simulink model "SimForces2020a"  (R2020a)
settings: Solver=daessc  StartTime=0.0  StopTime=10  FixedStep=0.001  RelTol=1e-4
values from neighbouring files (symbols this model uses):
  Bc1_V = [0;0;0;0;0;0]    [initializeSimulationGP.m]
  D22F = [0;0;0;0;0;0]    [initializeSimulationGP.m]
  filtDV = init2ndOrderLowPassFilter(35*2*pi,1,controller.dT)    [initializeLowPassFilters.m]
  filtEnc = init2ndOrderLowPassFilter(35*2*pi,1,controller.dT)    [initializeLowPassFilters.m]
undefined symbols (not defined in the file or in its folder): aux, B11_r_B11Tc1, B11_V, B11Ftot, B12_r_B12Tc2, B12_Rot_Tc2, B12_U_Tc2, B12_V, B12Ftot, B31_r_B31B41, B31_V, B31FTot, B32_r_B32B42, B32_Rot_B42, B32_U_B42, B32_V, B32FTot, B41_r_B41Tc1, B41_V, B41FTot, B42_r_B42Tc2, B42_Rot_Tc2, B42_U_Tc2, B42_V, B42FTot, B52_r_B52P32, B52_Rot_P32, B52_U_P32, B52_V, B52Ftot, Bc1_r_Bc1B11, Bc1_r_Bc1B31, Bc1FTot, Bc2_r_Bc2B12, Bc2_r_Bc2B32, Bc2_Rot_B12, Bc2_Rot_B32, Bc2_U_B12, Bc2_U_B32, Bc2_V, Bc2Tot, cmdMotion, controller, cyl1, cyl2, D22_V, dq1, dq11, dq12, dq2, dq21, dq22, dx1, dx2, dxt2, fc1, fc1r, fc2, fc2r, fct2 ... (+62)
libraries: sm_lib x31, nesl_utility x10
(part 4 of 7)

== system SimForces2020a/sbVDCController/sbFormTotalRequiredForces/sbTotalRequiredForcesRS1/sbFilteredVelocityDerivativeB11 ==
  u : Inport
  Demux : Demux  Outputs=6
  Mux : Mux  Inputs=6
  sbDiscreteDerivative1 : Subsystem
  sbDiscreteDerivative2 : Subsystem
  sbDiscreteDerivative3 : Subsystem
  sbDiscreteDerivative4 : Subsystem
  sbDiscreteDerivative5 : Subsystem
  sbDiscreteDerivative6 : Subsystem
  sbLowPassFilter1 : Subsystem
  sbLowPassFilter2 : Subsystem
  sbLowPassFilter3 : Subsystem
  sbLowPassFilter4 : Subsystem
  sbLowPassFilter5 : Subsystem
  sbLowPassFilter6 : Subsystem
  du : Outport
  wires:
  sbLowPassFilter5/1(dVFilt) -> Mux/5
  sbDiscreteDerivative4/1(du/dt) -> sbLowPassFilter4/1(dV)
  sbLowPassFilter4/1(dVFilt) -> Mux/4
  sbLowPassFilter3/1(dVFilt) -> Mux/3
  sbDiscreteDerivative3/1(du/dt) -> sbLowPassFilter3/1(dV)
  sbDiscreteDerivative2/1(du/dt) -> sbLowPassFilter2/1(dV)
  sbLowPassFilter6/1(dVFilt) -> Mux/6
  sbDiscreteDerivative6/1(du/dt) -> sbLowPassFilter6/1(dV)
  sbLowPassFilter1/1(dVFilt) -> Mux/1
  u/1 -> Demux/1
  Demux/2 -> sbDiscreteDerivative2/1(u)
  Demux/5 -> sbDiscreteDerivative5/1(u)
  sbDiscreteDerivative1/1(du/dt) -> sbLowPassFilter1/1(dV)
  Demux/6 -> sbDiscreteDerivative6/1(u)
  sbLowPassFilter2/1(dVFilt) -> Mux/2
  Demux/1 -> sbDiscreteDerivative1/1(u)
  Demux/4 -> sbDiscreteDerivative4/1(u)
  Mux/1 -> du/1
  sbDiscreteDerivative5/1(du/dt) -> sbLowPassFilter5/1(dV)
  Demux/3 -> sbDiscreteDerivative3/1(u)

== system SimForces2020a/sbVDCController/sbFormTotalRequiredForces/sbTotalRequiredForcesRS1/sbFilteredVelocityDerivativeB31 ==
  u : Inport
  Demux : Demux  Outputs=6
  Mux : Mux  Inputs=6
  sbDiscreteDerivative1 : Subsystem
  sbDiscreteDerivative2 : Subsystem
  sbDiscreteDerivative3 : Subsystem
  sbDiscreteDerivative4 : Subsystem
  sbDiscreteDerivative5 : Subsystem
  sbDiscreteDerivative6 : Subsystem
  sbLowPassFilter1 : Subsystem
  sbLowPassFilter2 : Subsystem
  sbLowPassFilter3 : Subsystem
  sbLowPassFilter4 : Subsystem
  sbLowPassFilter5 : Subsystem
  sbLowPassFilter6 : Subsystem
  du : Outport
  wires:
  Demux/3 -> sbDiscreteDerivative3/1(u)
  sbDiscreteDerivative5/1(du/dt) -> sbLowPassFilter5/1(dV)
  Mux/1 -> du/1
  Demux/4 -> sbDiscreteDerivative4/1(u)
  Demux/1 -> sbDiscreteDerivative1/1(u)
  sbLowPassFilter2/1(dVFilt) -> Mux/2
  Demux/6 -> sbDiscreteDerivative6/1(u)
  sbDiscreteDerivative1/1(du/dt) -> sbLowPassFilter1/1(dV)
  Demux/5 -> sbDiscreteDerivative5/1(u)
  Demux/2 -> sbDiscreteDerivative2/1(u)
  u/1 -> Demux/1
  sbLowPassFilter1/1(dVFilt) -> Mux/1
  sbDiscreteDerivative6/1(du/dt) -> sbLowPassFilter6/1(dV)
  sbLowPassFilter6/1(dVFilt) -> Mux/6
  sbDiscreteDerivative2/1(du/dt) -> sbLowPassFilter2/1(dV)
  sbDiscreteDerivative3/1(du/dt) -> sbLowPassFilter3/1(dV)
  sbLowPassFilter3/1(dVFilt) -> Mux/3
  sbLowPassFilter4/1(dVFilt) -> Mux/4
  sbDiscreteDerivative4/1(du/dt) -> sbLowPassFilter4/1(dV)
  sbLowPassFilter5/1(dVFilt) -> Mux/5

== system SimForces2020a/sbVDCController/sbFormTotalRequiredForces/sbTotalRequiredForcesRS1/sbFilteredVelocityDerivativeB41 ==
  u : Inport
  Demux : Demux  Outputs=6
  Mux : Mux  Inputs=6
  sbDiscreteDerivative1 : Subsystem
  sbDiscreteDerivative2 : Subsystem
  sbDiscreteDerivative3 : Subsystem
  sbDiscreteDerivative4 : Subsystem
  sbDiscreteDerivative5 : Subsystem
  sbDiscreteDerivative6 : Subsystem
  sbLowPassFilter1 : Subsystem
  sbLowPassFilter2 : Subsystem
  sbLowPassFilter3 : Subsystem
  sbLowPassFilter4 : Subsystem
  sbLowPassFilter5 : Subsystem
  sbLowPassFilter6 : Subsystem
  du : Outport
  wires:
  Demux/3 -> sbDiscreteDerivative3/1(u)
  sbDiscreteDerivative5/1(du/dt) -> sbLowPassFilter5/1(dV)
  Mux/1 -> du/1
  Demux/4 -> sbDiscreteDerivative4/1(u)
  Demux/1 -> sbDiscreteDerivative1/1(u)
  sbLowPassFilter2/1(dVFilt) -> Mux/2
  Demux/6 -> sbDiscreteDerivative6/1(u)
  sbDiscreteDerivative1/1(du/dt) -> sbLowPassFilter1/1(dV)
  Demux/5 -> sbDiscreteDerivative5/1(u)
  Demux/2 -> sbDiscreteDerivative2/1(u)
  u/1 -> Demux/1
  sbLowPassFilter1/1(dVFilt) -> Mux/1
  sbDiscreteDerivative6/1(du/dt) -> sbLowPassFilter6/1(dV)
  sbLowPassFilter6/1(dVFilt) -> Mux/6
  sbDiscreteDerivative2/1(du/dt) -> sbLowPassFilter2/1(dV)
  sbDiscreteDerivative3/1(du/dt) -> sbLowPassFilter3/1(dV)
  sbLowPassFilter3/1(dVFilt) -> Mux/3
  sbLowPassFilter4/1(dVFilt) -> Mux/4
  sbDiscreteDerivative4/1(du/dt) -> sbLowPassFilter4/1(dV)
  sbLowPassFilter5/1(dVFilt) -> Mux/5

== system SimForces2020a/sbVDCController/sbFormTotalRequiredForces/sbTotalRequiredForcesRS1/sbFilteredVelocityDerivativeBc1 ==
  u : Inport
  Demux : Demux  Outputs=6
  Mux : Mux  Inputs=6
  sbDiscreteDerivative1 : Subsystem
  sbDiscreteDerivative2 : Subsystem
  sbDiscreteDerivative3 : Subsystem
  sbDiscreteDerivative4 : Subsystem
  sbDiscreteDerivative5 : Subsystem
  sbDiscreteDerivative6 : Subsystem
  sbLowPassFilter1 : Subsystem
  sbLowPassFilter2 : Subsystem
  sbLowPassFilter3 : Subsystem
  sbLowPassFilter4 : Subsystem
  sbLowPassFilter5 : Subsystem
  sbLowPassFilter6 : Subsystem
  du : Outport
  wires:
  sbLowPassFilter5/1(dVFilt) -> Mux/5
  sbDiscreteDerivative4/1(du/dt) -> sbLowPassFilter4/1(dV)
  sbLowPassFilter4/1(dVFilt) -> Mux/4
  sbLowPassFilter3/1(dVFilt) -> Mux/3
  sbDiscreteDerivative3/1(du/dt) -> sbLowPassFilter3/1(dV)
  sbDiscreteDerivative2/1(du/dt) -> sbLowPassFilter2/1(dV)
  sbLowPassFilter6/1(dVFilt) -> Mux/6
  sbDiscreteDerivative6/1(du/dt) -> sbLowPassFilter6/1(dV)
  sbLowPassFilter1/1(dVFilt) -> Mux/1
  u/1 -> Demux/1
  Demux/2 -> sbDiscreteDerivative2/1(u)
  Demux/5 -> sbDiscreteDerivative5/1(u)
  sbDiscreteDerivative1/1(du/dt) -> sbLowPassFilter1/1(dV)
  Demux/6 -> sbDiscreteDerivative6/1(u)
  sbLowPassFilter2/1(dVFilt) -> Mux/2
  Demux/1 -> sbDiscreteDerivative1/1(u)
  Demux/4 -> sbDiscreteDerivative4/1(u)
  Mux/1 -> du/1
  sbDiscreteDerivative5/1(du/dt) -> sbLowPassFilter5/1(dV)
  Demux/3 -> sbDiscreteDerivative3/1(u)

== system SimForces2020a/sbVDCController/sbFormTotalRequiredForces/sbTotalRequiredForcesRS2/sbFilteredVelocityDerivativeB12 ==
  u : Inport
  Demux : Demux  Outputs=6
  Mux : Mux  Inputs=6
  sbDiscreteDerivative1 : Subsystem
  sbDiscreteDerivative2 : Subsystem
  sbDiscreteDerivative3 : Subsystem
  sbDiscreteDerivative4 : Subsystem
  sbDiscreteDerivative5 : Subsystem
  sbDiscreteDerivative6 : Subsystem
  sbLowPassFilter1 : Subsystem
  sbLowPassFilter2 : Subsystem
  sbLowPassFilter3 : Subsystem
  sbLowPassFilter4 : Subsystem
  sbLowPassFilter5 : Subsystem
  sbLowPassFilter6 : Subsystem
  du : Outport
  wires:
  Demux/3 -> sbDiscreteDerivative3/1(u)
  sbDiscreteDerivative5/1(du/dt) -> sbLowPassFilter5/1(dV)
  Mux/1 -> du/1
  Demux/4 -> sbDiscreteDerivative4/1(u)
  Demux/1 -> sbDiscreteDerivative1/1(u)
  sbLowPassFilter2/1(dVFilt) -> Mux/2
  Demux/6 -> sbDiscreteDerivative6/1(u)
  sbDiscreteDerivative1/1(du/dt) -> sbLowPassFilter1/1(dV)
  Demux/5 -> sbDiscreteDerivative5/1(u)
  Demux/2 -> sbDiscreteDerivative2/1(u)
  u/1 -> Demux/1
  sbLowPassFilter1/1(dVFilt) -> Mux/1
  sbDiscreteDerivative6/1(du/dt) -> sbLowPassFilter6/1(dV)
  sbLowPassFilter6/1(dVFilt) -> Mux/6
  sbDiscreteDerivative2/1(du/dt) -> sbLowPassFilter2/1(dV)
  sbDiscreteDerivative3/1(du/dt) -> sbLowPassFilter3/1(dV)
  sbLowPassFilter3/1(dVFilt) -> Mux/3
  sbLowPassFilter4/1(dVFilt) -> Mux/4
  sbDiscreteDerivative4/1(du/dt) -> sbLowPassFilter4/1(dV)
  sbLowPassFilter5/1(dVFilt) -> Mux/5

== system SimForces2020a/sbVDCController/sbFormTotalRequiredForces/sbTotalRequiredForcesRS2/sbFilteredVelocityDerivativeB32 ==
  u : Inport
  Demux : Demux  Outputs=6
  Mux : Mux  Inputs=6
  sbDiscreteDerivative1 : Subsystem
  sbDiscreteDerivative2 : Subsystem
  sbDiscreteDerivative3 : Subsystem
  sbDiscreteDerivative4 : Subsystem
  sbDiscreteDerivative5 : Subsystem
  sbDiscreteDerivative6 : Subsystem
  sbLowPassFilter1 : Subsystem
  sbLowPassFilter2 : Subsystem
  sbLowPassFilter3 : Subsystem
  sbLowPassFilter4 : Subsystem
  sbLowPassFilter5 : Subsystem
  sbLowPassFilter6 : Subsystem
  du : Outport
  wires:
  Demux/3 -> sbDiscreteDerivative3/1(u)
  sbDiscreteDerivative5/1(du/dt) -> sbLowPassFilter5/1(dV)
  Mux/1 -> du/1
  Demux/4 -> sbDiscreteDerivative4/1(u)
  Demux/1 -> sbDiscreteDerivative1/1(u)
  sbLowPassFilter2/1(dVFilt) -> Mux/2
  Demux/6 -> sbDiscreteDerivative6/1(u)
  sbDiscreteDerivative1/1(du/dt) -> sbLowPassFilter1/1(dV)
  Demux/5 -> sbDiscreteDerivative5/1(u)
  Demux/2 -> sbDiscreteDerivative2/1(u)
  u/1 -> Demux/1
  sbLowPassFilter1/1(dVFilt) -> Mux/1
  sbDiscreteDerivative6/1(du/dt) -> sbLowPassFilter6/1(dV)
  sbLowPassFilter6/1(dVFilt) -> Mux/6
  sbDiscreteDerivative2/1(du/dt) -> sbLowPassFilter2/1(dV)
  sbDiscreteDerivative3/1(du/dt) -> sbLowPassFilter3/1(dV)
  sbLowPassFilter3/1(dVFilt) -> Mux/3
  sbLowPassFilter4/1(dVFilt) -> Mux/4
  sbDiscreteDerivative4/1(du/dt) -> sbLowPassFilter4/1(dV)
  sbLowPassFilter5/1(dVFilt) -> Mux/5

== system SimForces2020a/sbVDCController/sbFormTotalRequiredForces/sbTotalRequiredForcesRS2/sbFilteredVelocityDerivativeB42 ==
  u : Inport
  Demux : Demux  Outputs=6
  Mux : Mux  Inputs=6
  sbDiscreteDerivative1 : Subsystem
  sbDiscreteDerivative2 : Subsystem
  sbDiscreteDerivative3 : Subsystem
  sbDiscreteDerivative4 : Subsystem
  sbDiscreteDerivative5 : Subsystem
  sbDiscreteDerivative6 : Subsystem
  sbLowPassFilter1 : Subsystem
  sbLowPassFilter2 : Subsystem
  sbLowPassFilter3 : Subsystem
  sbLowPassFilter4 : Subsystem
  sbLowPassFilter5 : Subsystem
  sbLowPassFilter6 : Subsystem
  du : Outport
  wires:
  Demux/3 -> sbDiscreteDerivative3/1(u)
  sbDiscreteDerivative5/1(du/dt) -> sbLowPassFilter5/1(dV)
  Mux/1 -> du/1
  Demux/4 -> sbDiscreteDerivative4/1(u)
  Demux/1 -> sbDiscreteDerivative1/1(u)
  sbLowPassFilter2/1(dVFilt) -> Mux/2
  Demux/6 -> sbDiscreteDerivative6/1(u)
  sbDiscreteDerivative1/1(du/dt) -> sbLowPassFilter1/1(dV)
  Demux/5 -> sbDiscreteDerivative5/1(u)
  Demux/2 -> sbDiscreteDerivative2/1(u)
  u/1 -> Demux/1
  sbLowPassFilter1/1(dVFilt) -> Mux/1
  sbDiscreteDerivative6/1(du/dt) -> sbLowPassFilter6/1(dV)
  sbLowPassFilter6/1(dVFilt) -> Mux/6
  sbDiscreteDerivative2/1(du/dt) -> sbLowPassFilter2/1(dV)
  sbDiscreteDerivative3/1(du/dt) -> sbLowPassFilter3/1(dV)
  sbLowPassFilter3/1(dVFilt) -> Mux/3
  sbLowPassFilter4/1(dVFilt) -> Mux/4
  sbDiscreteDerivative4/1(du/dt) -> sbLowPassFilter4/1(dV)
  sbLowPassFilter5/1(dVFilt) -> Mux/5

== system SimForces2020a/sbVDCController/sbFormTotalRequiredForces/sbTotalRequiredForcesRS2/sbFilteredVelocityDerivativeBc2 ==
  u : Inport
  Demux : Demux  Outputs=6
  Mux : Mux  Inputs=6
  sbDiscreteDerivative1 : Subsystem
  sbDiscreteDerivative2 : Subsystem
  sbDiscreteDerivative3 : Subsystem
  sbDiscreteDerivative4 : Subsystem
  sbDiscreteDerivative5 : Subsystem
  sbDiscreteDerivative6 : Subsystem
  sbLowPassFilter1 : Subsystem
  sbLowPassFilter2 : Subsystem
  sbLowPassFilter3 : Subsystem
  sbLowPassFilter4 : Subsystem
  sbLowPassFilter5 : Subsystem
  sbLowPassFilter6 : Subsystem
  du : Outport
  wires:
  Demux/3 -> sbDiscreteDerivative3/1(u)
  sbDiscreteDerivative5/1(du/dt) -> sbLowPassFilter5/1(dV)
  Mux/1 -> du/1
  Demux/4 -> sbDiscreteDerivative4/1(u)
  Demux/1 -> sbDiscreteDerivative1/1(u)
  sbLowPassFilter2/1(dVFilt) -> Mux/2
  Demux/6 -> sbDiscreteDerivative6/1(u)
  sbDiscreteDerivative1/1(du/dt) -> sbLowPassFilter1/1(dV)
  Demux/5 -> sbDiscreteDerivative5/1(u)
  Demux/2 -> sbDiscreteDerivative2/1(u)
  u/1 -> Demux/1
  sbLowPassFilter1/1(dVFilt) -> Mux/1
  sbDiscreteDerivative6/1(du/dt) -> sbLowPassFilter6/1(dV)
  sbLowPassFilter6/1(dVFilt) -> Mux/6
  sbDiscreteDerivative2/1(du/dt) -> sbLowPassFilter2/1(dV)
  sbDiscreteDerivative3/1(du/dt) -> sbLowPassFilter3/1(dV)
  sbLowPassFilter3/1(dVFilt) -> Mux/3
  sbLowPassFilter4/1(dVFilt) -> Mux/4
  sbDiscreteDerivative4/1(du/dt) -> sbLowPassFilter4/1(dV)
  sbLowPassFilter5/1(dVFilt) -> Mux/5

== system SimForces2020a/sbVDCController/sbFormAnalyticQuantities/sbPrismaticSegment2/sbGeomPropPS2/sbDiscreteDerivative ==
  u : Inport
  Add : Sum  Inputs=-+
  Gain6 : Gain  Gain=1/(2*controller.dT)
  Integer Delay : Delay  InitialConditionSource=Input port  InitialCondition=0  SampleTime=controller.dT
      settings: InputPortMap=u0,p4
  du/dt : Outport  PortDimensions=1
  wires:
  u/1 -> Integer Delay/1, Integer Delay/2, Add/2
  Gain6/1 -> du/dt/1
  Integer Delay/1 -> Add/1
  Add/1 -> Gain6/1

== system SimForces2020a/sbVDCController/sbFormAnalyticQuantities/sbRevoluteSegment1/sbGeomPropRS1/sbLiftPistonStroke ==
  note: Get inputs...
  note: Process data...
  note: Pass to outputs...
  q1 : Inport  Unit=rad  PortDimensions=1
  liftPistonStroke : MATLAB Function  TreatAsAtomicUnit=on
  x1 : Outport  Unit=m  PortDimensions=1
  wires:
  [x1] -> x1/1  "x1"
  liftPistonStroke/1(x1) -> [x1]  "x1"
  [q1] -> liftPistonStroke/1(q1)  "q1"
  q1/1 -> [q1]  "q1"

== system SimForces2020a/sbVDCController/sbFormAnalyticQuantities/sbRevoluteSegment1/sbGeomPropRS1/sbLiftPistonVelocity ==
  note: Get inputs...
  note: Process data...
  note: Pass to output...
  dq1 : Inport
  x1 : Inport  Port=2
  q1 : Inport  Port=3
  liftPistonVelocity : MATLAB Function  TreatAsAtomicUnit=on
  dx1 : Outport
  wires:
  [dx1] -> dx1/1  "dx1"
  liftPistonVelocity/1(dx1) -> [dx1]  "dx1"
  [q1] -> liftPistonVelocity/3(q1)  "q1"
  q1/1 -> [q1]  "q1"
  [x1] -> liftPistonVelocity/2(x1)  "x1"
  x1/1 -> [x1]  "x1"
  [dq1] -> liftPistonVelocity/1(dq1)  "dq1"
  dq1/1 -> [dq1]  "dq1"

== system SimForces2020a/sbVDCController/sbFormAnalyticQuantities/sbRevoluteSegment1/sbGeomPropRS1/sbq11AngleValue ==
  note: Get inputs...
  note: Process data...
  note: Pass to outputs...
  x1 : Inport
  q11AngleValue : MATLAB Function  TreatAsAtomicUnit=on
  q11 : Outport
  wires:
  [q11] -> q11/1  "q11"
  q11AngleValue/1(q11) -> [q11]  "q11"
  [x1] -> q11AngleValue/1(x1)  "x1"
  x1/1 -> [x1]  "x1"

== system SimForces2020a/sbVDCController/sbFormAnalyticQuantities/sbRevoluteSegment1/sbGeomPropRS1/sbq11AngleVelocity ==
  note: Get inputs...
  note: Process data...
  note: Pass to outputs...
  x1 : Inport
  q11 : Inport  Port=2
  dx1 : Inport  Port=3
  q11AngleRate : MATLAB Function  TreatAsAtomicUnit=on
  dq11 : Outport
  wires:
  [dq11] -> dq11/1  "dq11"
  q11AngleRate/1(dq11) -> [dq11]  "dq11"
  [dx1] -> q11AngleRate/3(dx1)  "dx1"
  [q11] -> q11AngleRate/2(q11)  "q11"
  [x1] -> q11AngleRate/1(x1)  "x1"
  dx1/1 -> [dx1]  "dx1"
  q11/1 -> [q11]  "q11"
  x1/1 -> [x1]  "x1"

== system SimForces2020a/sbVDCController/sbFormAnalyticQuantities/sbRevoluteSegment1/sbGeomPropRS1/sbq12AngleRate ==
  note: Get inputs...
  note: Pass to outputs...
  note: Process data...
  x1 : Inport
  q12 : Inport  Port=2
  dx1 : Inport  Port=3
  q12AngleRate : MATLAB Function  TreatAsAtomicUnit=on
  dq12 : Outport
  wires:
  [dx1] -> q12AngleRate/3(dx1)  "dx1"
  [x1] -> q12AngleRate/1(x1)  "x1"
  [q12] -> q12AngleRate/2(q12)  "q12"
  x1/1 -> [x1]  "x1"
  q12AngleRate/1(dq12) -> [dq12]  "dq12"
  [dq12] -> dq12/1  "dq12"
  q12/1 -> [q12]  "q12"
  dx1/1 -> [dx1]  "dx1"

== system SimForces2020a/sbVDCController/sbFormAnalyticQuantities/sbRevoluteSegment1/sbGeomPropRS1/sbq12AngleValue ==
  note: Get inputs...
  note: Process data...
  note: Pass to outputs...
  x1 : Inport
  q12AngleValue : MATLAB Function  TreatAsAtomicUnit=on
  q12 : Outport
  wires:
  [q12] -> q12/1  "q12"
  q12AngleValue/1(q12) -> [q12]  "q12"
  [x1] -> q12AngleValue/1(x1)  "x1"
  x1/1 -> [x1]  "x1"

== system SimForces2020a/sbVDCController/sbFormAnalyticQuantities/sbRevoluteSegment1/sbGeomPropRS1/sbq1AngleRate ==
  note: Get inputs...
  note: Process data...
  note: Pass to outputs...
  q1 : Inport
  sbDiscreteDerivative : Subsystem
  dq1 : Outport
  wires:
  sbDiscreteDerivative/1(du/dt) -> [dq1]  "dq1"
  [dq1] -> dq1/1  "dq1"
  [q1] -> sbDiscreteDerivative/1(u)  "q1"
  q1/1 -> [q1]  "q1"

== system SimForces2020a/sbVDCController/sbFormAnalyticQuantities/sbRevoluteSegment2/sbGeomPropRS2/sbTiltPistonStroke ==
  note: Pass to outputs...
  note: Get inputs...
  note: Derive the tilt piston stroke from q2-angle value...
  note: Process data...
  q2 : Inport
  tiltPistonStroke : MATLAB Function  TreatAsAtomicUnit=on
  x2 : Outport
  wires:
  q2/1 -> [q2]  "q2"
  [x2] -> x2/1  "x2"
  tiltPistonStroke/1(x2) -> [x2]  "x2"
  [q2] -> tiltPistonStroke/1(q2)  "q2"

== system SimForces2020a/sbVDCController/sbFormAnalyticQuantities/sbRevoluteSegment2/sbGeomPropRS2/sbTiltPistonVelocity ==
  note: Get inputs...
  note: Process data...
  note: Pass to output...
  dq2 : Inport
  x2 : Inport  Port=2
  q2 : Inport  Port=3
  tiltPistonVelocity : MATLAB Function  TreatAsAtomicUnit=on
  dx2 : Outport
  wires:
  tiltPistonVelocity/1(dx2) -> [dx2]  "dx2"
  [dx2] -> dx2/1  "dx2"
  [q2] -> tiltPistonVelocity/3(q2)  "q2"
  q2/1 -> [q2]  "q2"
  [x2] -> tiltPistonVelocity/2(x2)  "x2"
  x2/1 -> [x2]  "x2"
  [dq2] -> tiltPistonVelocity/1(dq2)  "dq2"
  dq2/1 -> [dq2]  "dq2"

== system SimForces2020a/sbVDCController/sbFormAnalyticQuantities/sbRevoluteSegment2/sbGeomPropRS2/sbq21AngleRate ==
  note: Get inputs...
  note: Process data...
  note: Pass to outputs...
  x2 : Inport
  q21 : Inport  Port=2
  dx2 : Inport  Port=3
  q21AngleRate : MATLAB Function  TreatAsAtomicUnit=on
  dq21 : Outport
  wires:
  [q21] -> q21AngleRate/2(q21)  "q21"
  [dx2] -> q21AngleRate/3(dx2)  "dx2"
  [dq21] -> dq21/1  "dq21"
  q21AngleRate/1(dq21) -> [dq21]  "dq21"
  [x2] -> q21AngleRate/1(x2)  "x2"
  dx2/1 -> [dx2]  "dx2"
  q21/1 -> [q21]  "q21"
  x2/1 -> [x2]  "x2"

== system SimForces2020a/sbVDCController/sbFormAnalyticQuantities/sbRevoluteSegment2/sbGeomPropRS2/sbq21AngleValue ==
  note: Get inputs...
  note: Process data...
  note: Pass to outputs...
  x2 : Inport
  q21AngleValue : MATLAB Function  TreatAsAtomicUnit=on
  q21 : Outport
  wires:
  q21AngleValue/1(q21) -> [q21]  "q21"
  [x2] -> q21AngleValue/1(x2)  "x2"
  [q21] -> q21/1  "q21"
  x2/1 -> [x2]  "x2"

== system SimForces2020a/sbVDCController/sbFormAnalyticQuantities/sbRevoluteSegment2/sbGeomPropRS2/sbq22AngleRate ==
  note: Get inputs...
  note: Pass to outputs...
  note: Process data...
  x2 : Inport
  q22 : Inport  Port=2
  dx2 : Inport  Port=3
  q22AngleRate : MATLAB Function  TreatAsAtomicUnit=on
  dq22 : Outport
  wires:
  [x2] -> q22AngleRate/1(x2)  "x2"
  x2/1 -> [x2]  "x2"
  q22AngleRate/1(dq22) -> [dq22]  "dq22"
  [dq22] -> dq22/1  "dq22"
  q22/1 -> [q22]  "q22"
  dx2/1 -> [dx2]  "dx2"
  [q22] -> q22AngleRate/2(q22)  "q22"
  [dx2] -> q22AngleRate/3(dx2)  "dx2"

== system SimForces2020a/sbVDCController/sbFormAnalyticQuantities/sbRevoluteSegment2/sbGeomPropRS2/sbq22AngleValue ==
  note: Pass to outputs...
  note: Process data...
  note: Get inputs...
  x2 : Inport
  q22AngleValue : MATLAB Function  TreatAsAtomicUnit=on
  q22 : Outport
  wires:
  x2/1 -> [x2]  "x2"
  [x2] -> q22AngleValue/1(x2)  "x2"
  q22AngleValue/1(q22) -> [q22]  "q22"
  [q22] -> q22/1  "q22"

== system SimForces2020a/sbVDCController/sbFormAnalyticQuantities/sbRevoluteSegment2/sbGeomPropRS2/sbq2AngleRate ==
  note: Get inputs...
  note: Process data...
  note: Pass to outputs...
  q2 : Inport
  sbDiscreteDerivative : Subsystem
  dq2 : Outport
  wires:
  sbDiscreteDerivative/1(du/dt) -> [dq2]  "dq2"
  [dq2] -> dq2/1  "dq2"
  [q2] -> sbDiscreteDerivative/1(u)  "q2"
  q2/1 -> [q2]  "q2"

== system SimForces2020a/sbVDCController/sbFormTotalRequiredForces/sbTotalRequiredForcesPS2/sbFilteredVelocityDerivativeB52/sbDiscreteDerivative1 ==
  u : Inport
  Add : Sum  Inputs=-+
  Gain6 : Gain  Gain=1/(2*controller.dT)
  Integer Delay : Delay  InitialConditionSource=Input port  InitialCondition=0  SampleTime=controller.dT
      settings: InputPortMap=u0,p4
  du/dt : Outport  PortDimensions=1
  wires:
  Add/1 -> Gain6/1
  u/1 -> Integer Delay/1, Integer Delay/2, Add/2
  Integer Delay/1 -> Add/1
  Gain6/1 -> du/dt/1

== system SimForces2020a/sbVDCController/sbFormTotalRequiredForces/sbTotalRequiredForcesPS2/sbFilteredVelocityDerivativeB52/sbDiscreteDerivative2 ==
  u : Inport
  Add : Sum  Inputs=-+
  Gain6 : Gain  Gain=1/(2*controller.dT)
  Integer Delay : Delay  InitialConditionSource=Input port  InitialCondition=0  SampleTime=controller.dT
      settings: InputPortMap=u0,p4
  du/dt : Outport  PortDimensions=1
  wires:
  u/1 -> Integer Delay/1, Integer Delay/2, Add/2
  Integer Delay/1 -> Add/1
  Add/1 -> Gain6/1
  Gain6/1 -> du/dt/1

== system SimForces2020a/sbVDCController/sbFormTotalRequiredForces/sbTotalRequiredForcesPS2/sbFilteredVelocityDerivativeB52/sbDiscreteDerivative3 ==
  u : Inport
  Add : Sum  Inputs=-+
  Gain6 : Gain  Gain=1/(2*controller.dT)
  Integer Delay : Delay  InitialConditionSource=Input port  InitialCondition=0  SampleTime=controller.dT
      settings: InputPortMap=u0,p4
  du/dt : Outport  PortDimensions=1
  wires:
  Add/1 -> Gain6/1
  Integer Delay/1 -> Add/1
  u/1 -> Integer Delay/1, Integer Delay/2, Add/2
  Gain6/1 -> du/dt/1

== system SimForces2020a/sbVDCController/sbFormTotalRequiredForces/sbTotalRequiredForcesPS2/sbFilteredVelocityDerivativeB52/sbDiscreteDerivative4 ==
  u : Inport
  Add : Sum  Inputs=-+
  Gain6 : Gain  Gain=1/(2*controller.dT)
  Integer Delay : Delay  InitialConditionSource=Input port  InitialCondition=0  SampleTime=controller.dT
      settings: InputPortMap=u0,p4
  du/dt : Outport  PortDimensions=1
  wires:
  Add/1 -> Gain6/1
  Integer Delay/1 -> Add/1
  u/1 -> Integer Delay/1, Integer Delay/2, Add/2
  Gain6/1 -> du/dt/1

== system SimForces2020a/sbVDCController/sbFormTotalRequiredForces/sbTotalRequiredForcesPS2/sbFilteredVelocityDerivativeB52/sbDiscreteDerivative5 ==
  u : Inport
  Add : Sum  Inputs=-+
  Gain6 : Gain  Gain=1/(2*controller.dT)
  Integer Delay : Delay  InitialConditionSource=Input port  InitialCondition=0  SampleTime=controller.dT
      settings: InputPortMap=u0,p4
  du/dt : Outport  PortDimensions=1
  wires:
  Add/1 -> Gain6/1
  Integer Delay/1 -> Add/1
  u/1 -> Integer Delay/1, Integer Delay/2, Add/2
  Gain6/1 -> du/dt/1

== system SimForces2020a/sbVDCController/sbFormTotalRequiredForces/sbTotalRequiredForcesPS2/sbFilteredVelocityDerivativeB52/sbDiscreteDerivative6 ==
  u : Inport
  Add : Sum  Inputs=-+
  Gain6 : Gain  Gain=1/(2*controller.dT)
  Integer Delay : Delay  InitialConditionSource=Input port  InitialCondition=0  SampleTime=controller.dT
      settings: InputPortMap=u0,p4
  du/dt : Outport  PortDimensions=1
  wires:
  Add/1 -> Gain6/1
  Integer Delay/1 -> Add/1
  u/1 -> Integer Delay/1, Integer Delay/2, Add/2
  Gain6/1 -> du/dt/1

== system SimForces2020a/sbVDCController/sbFormTotalRequiredForces/sbTotalRequiredForcesPS2/sbFilteredVelocityDerivativeB52/sbLowPassFilter1 ==
  dV : Inport
  Delay : Delay  InitialConditionSource=Input port  SampleTime=filtDV.dT
      settings: InputPortMap=u0,p4
  Delay1 : Delay  DelayLength=1  InitialConditionSource=Input port  SampleTime=filtDV.dT
      settings: InputPortMap=u0,p4
  Delay2 : Delay  DelayLength=0  InitialConditionSource=Input port  SampleTime=filtDV.dT
      settings: InputPortMap=u0,p4
  Delay3 : Delay  InitialConditionSource=Input port  SampleTime=filtDV.dT
      settings: InputPortMap=u0,p4
  Delay4 : Delay  DelayLength=1  InitialConditionSource=Input port  SampleTime=filtDV.dT
      settings: InputPortMap=u0,p4
  Gain : Gain  Gain=filtDV.a0
  Gain1 : Gain  Gain=filtDV.b1
  Gain2 : Gain  Gain=filtDV.b2
  Gain3 : Gain  Gain=filtDV.b0
  Gain4 : Gain  Gain=filtDV.a1
  Sum : Sum  Inputs=|--+++
  dVFilt : Outport
  wires:
  Gain3/1 -> Sum/5
  Gain2/1 -> Sum/3
  Delay4/1 -> Gain4/1
  Delay/1 -> Gain/1
  Delay1/1 -> Gain1/1
  Delay2/1 -> Gain2/1
  Gain4/1 -> Sum/1
  Sum/1 -> dVFilt/1, Delay4/1, Delay/1  "dVFilt"
  dV/1 -> Delay2/1, Delay2/2, Delay1/1, Delay3/2, Delay3/1, Delay1/2, Delay4/2, Delay/2  "dV"
  Gain1/1 -> Sum/4
  Gain/1 -> Sum/2
  Delay3/1 -> Gain3/1

== system SimForces2020a/sbVDCController/sbFormTotalRequiredForces/sbTotalRequiredForcesPS2/sbFilteredVelocityDerivativeB52/sbLowPassFilter2 ==
  dV : Inport
  Delay : Delay  InitialConditionSource=Input port  SampleTime=filtDV.dT
      settings: InputPortMap=u0,p4
  Delay1 : Delay  DelayLength=1  InitialConditionSource=Input port  SampleTime=filtDV.dT
      settings: InputPortMap=u0,p4
  Delay2 : Delay  DelayLength=0  InitialConditionSource=Input port  SampleTime=filtDV.dT
      settings: InputPortMap=u0,p4
  Delay3 : Delay  InitialConditionSource=Input port  SampleTime=filtDV.dT
      settings: InputPortMap=u0,p4
  Delay4 : Delay  DelayLength=1  InitialConditionSource=Input port  SampleTime=filtDV.dT
      settings: InputPortMap=u0,p4
  Gain : Gain  Gain=filtDV.a0
  Gain1 : Gain  Gain=filtDV.b1
  Gain2 : Gain  Gain=filtDV.b2
  Gain3 : Gain  Gain=filtDV.b0
  Gain4 : Gain  Gain=filtDV.a1
  Sum : Sum  Inputs=|--+++
  dVFilt : Outport
  wires:
  Delay3/1 -> Gain3/1
  Gain/1 -> Sum/2
  Gain1/1 -> Sum/4
  dV/1 -> Delay/2, Delay4/2, Delay1/2, Delay3/1, Delay3/2, Delay1/1, Delay2/2, Delay2/1  "dV"
  Sum/1 -> Delay/1, Delay4/1, dVFilt/1  "dVFilt"
  Gain4/1 -> Sum/1
  Delay2/1 -> Gain2/1
  Delay1/1 -> Gain1/1
  Delay/1 -> Gain/1
  Delay4/1 -> Gain4/1
  Gain2/1 -> Sum/3
  Gain3/1 -> Sum/5

== system SimForces2020a/sbVDCController/sbFormTotalRequiredForces/sbTotalRequiredForcesPS2/sbFilteredVelocityDerivativeB52/sbLowPassFilter3 ==
  dV : Inport
  Delay : Delay  InitialConditionSource=Input port  SampleTime=filtDV.dT
      settings: InputPortMap=u0,p4
  Delay1 : Delay  DelayLength=1  InitialConditionSource=Input port  SampleTime=filtDV.dT
      settings: InputPortMap=u0,p4
  Delay2 : Delay  DelayLength=0  InitialConditionSource=Input port  SampleTime=filtDV.dT
      settings: InputPortMap=u0,p4
  Delay3 : Delay  InitialConditionSource=Input port  SampleTime=filtDV.dT
      settings: InputPortMap=u0,p4
  Delay4 : Delay  DelayLength=1  InitialConditionSource=Input port  SampleTime=filtDV.dT
      settings: InputPortMap=u0,p4
  Gain : Gain  Gain=filtDV.a0
  Gain1 : Gain  Gain=filtDV.b1
  Gain2 : Gain  Gain=filtDV.b2
  Gain3 : Gain  Gain=filtDV.b0
  Gain4 : Gain  Gain=filtDV.a1
  Sum : Sum  Inputs=|--+++
  dVFilt : Outport
  wires:
  Gain3/1 -> Sum/5
  Gain2/1 -> Sum/3
  Delay4/1 -> Gain4/1
  Delay/1 -> Gain/1
  Delay1/1 -> Gain1/1
  Delay2/1 -> Gain2/1
  Gain4/1 -> Sum/1
  Sum/1 -> dVFilt/1, Delay4/1, Delay/1  "dVFilt"
  dV/1 -> Delay2/1, Delay2/2, Delay1/1, Delay3/2, Delay3/1, Delay1/2, Delay4/2, Delay/2  "dV"
  Gain1/1 -> Sum/4
  Gain/1 -> Sum/2
  Delay3/1 -> Gain3/1

== system SimForces2020a/sbVDCController/sbFormTotalRequiredForces/sbTotalRequiredForcesPS2/sbFilteredVelocityDerivativeB52/sbLowPassFilter4 ==
  dV : Inport
  Delay : Delay  InitialConditionSource=Input port  SampleTime=filtDV.dT
      settings: InputPortMap=u0,p4
  Delay1 : Delay  DelayLength=1  InitialConditionSource=Input port  SampleTime=filtDV.dT
      settings: InputPortMap=u0,p4
  Delay2 : Delay  DelayLength=0  InitialConditionSource=Input port  SampleTime=filtDV.dT
      settings: InputPortMap=u0,p4
  Delay3 : Delay  InitialConditionSource=Input port  SampleTime=filtDV.dT
      settings: InputPortMap=u0,p4
  Delay4 : Delay  DelayLength=1  InitialConditionSource=Input port  SampleTime=filtDV.dT
      settings: InputPortMap=u0,p4
  Gain : Gain  Gain=filtDV.a0
  Gain1 : Gain  Gain=filtDV.b1
  Gain2 : Gain  Gain=filtDV.b2
  Gain3 : Gain  Gain=filtDV.b0
  Gain4 : Gain  Gain=filtDV.a1
  Sum : Sum  Inputs=|--+++
  dVFilt : Outport
  wires:
  Delay3/1 -> Gain3/1
  Gain/1 -> Sum/2
  Gain1/1 -> Sum/4
  dV/1 -> Delay/2, Delay4/2, Delay1/2, Delay3/1, Delay3/2, Delay1/1, Delay2/2, Delay2/1  "dV"
  Sum/1 -> Delay/1, Delay4/1, dVFilt/1  "dVFilt"
  Gain4/1 -> Sum/1
  Delay2/1 -> Gain2/1
  Delay1/1 -> Gain1/1
  Delay/1 -> Gain/1
  Delay4/1 -> Gain4/1
  Gain2/1 -> Sum/3
  Gain3/1 -> Sum/5

== system SimForces2020a/sbVDCController/sbFormTotalRequiredForces/sbTotalRequiredForcesPS2/sbFilteredVelocityDerivativeB52/sbLowPassFilter5 ==
  dV : Inport
  Delay : Delay  InitialConditionSource=Input port  SampleTime=filtDV.dT
      settings: InputPortMap=u0,p4
  Delay1 : Delay  DelayLength=1  InitialConditionSource=Input port  SampleTime=filtDV.dT
      settings: InputPortMap=u0,p4
  Delay2 : Delay  DelayLength=0  InitialConditionSource=Input port  SampleTime=filtDV.dT
      settings: InputPortMap=u0,p4
  Delay3 : Delay  InitialConditionSource=Input port  SampleTime=filtDV.dT
      settings: InputPortMap=u0,p4
  Delay4 : Delay  DelayLength=1  InitialConditionSource=Input port  SampleTime=filtDV.dT
      settings: InputPortMap=u0,p4
  Gain : Gain  Gain=filtDV.a0
  Gain1 : Gain  Gain=filtDV.b1
  Gain2 : Gain  Gain=filtDV.b2
  Gain3 : Gain  Gain=filtDV.b0
  Gain4 : Gain  Gain=filtDV.a1
  Sum : Sum  Inputs=|--+++
  dVFilt : Outport
  wires:
  Gain3/1 -> Sum/5
  Gain2/1 -> Sum/3
  Delay4/1 -> Gain4/1
  Delay/1 -> Gain/1
  Delay1/1 -> Gain1/1
  Delay2/1 -> Gain2/1
  Gain4/1 -> Sum/1
  Sum/1 -> dVFilt/1, Delay4/1, Delay/1  "dVFilt"
  dV/1 -> Delay2/1, Delay2/2, Delay1/1, Delay3/2, Delay3/1, Delay1/2, Delay4/2, Delay/2  "dV"
  Gain1/1 -> Sum/4
  Gain/1 -> Sum/2
  Delay3/1 -> Gain3/1

== system SimForces2020a/sbVDCController/sbFormTotalRequiredForces/sbTotalRequiredForcesPS2/sbFilteredVelocityDerivativeB52/sbLowPassFilter6 ==
  dV : Inport
  Delay : Delay  InitialConditionSource=Input port  SampleTime=filtDV.dT
      settings: InputPortMap=u0,p4
  Delay1 : Delay  DelayLength=1  InitialConditionSource=Input port  SampleTime=filtDV.dT
      settings: InputPortMap=u0,p4
  Delay2 : Delay  DelayLength=0  InitialConditionSource=Input port  SampleTime=filtDV.dT
      settings: InputPortMap=u0,p4
  Delay3 : Delay  InitialConditionSource=Input port  SampleTime=filtDV.dT
      settings: InputPortMap=u0,p4
  Delay4 : Delay  DelayLength=1  InitialConditionSource=Input port  SampleTime=filtDV.dT
      settings: InputPortMap=u0,p4
  Gain : Gain  Gain=filtDV.a0
  Gain1 : Gain  Gain=filtDV.b1
  Gain2 : Gain  Gain=filtDV.b2
  Gain3 : Gain  Gain=filtDV.b0
  Gain4 : Gain  Gain=filtDV.a1
  Sum : Sum  Inputs=|--+++
  dVFilt : Outport
  wires:
  Delay3/1 -> Gain3/1
  Gain/1 -> Sum/2
  Gain1/1 -> Sum/4
  dV/1 -> Delay/2, Delay4/2, Delay1/2, Delay3/1, Delay3/2, Delay1/1, Delay2/2, Delay2/1  "dV"
  Sum/1 -> Delay/1, Delay4/1, dVFilt/1  "dVFilt"
  Gain4/1 -> Sum/1
  Delay2/1 -> Gain2/1
  Delay1/1 -> Gain1/1
  Delay/1 -> Gain/1
  Delay4/1 -> Gain4/1
  Gain2/1 -> Sum/3
  Gain3/1 -> Sum/5

== system SimForces2020a/sbVDCController/sbFormTotalRequiredForces/sbTotalRequiredForcesPS2/sbFilteredVelocityDerivativeP22/sbDiscreteDerivative1 ==
  u : Inport
  Add : Sum  Inputs=-+
  Gain6 : Gain  Gain=1/(2*controller.dT)
  Integer Delay : Delay  InitialConditionSource=Input port  InitialCondition=0  SampleTime=controller.dT
      settings: InputPortMap=u0,p4
  du/dt : Outport  PortDimensions=1
  wires:
  Add/1 -> Gain6/1
  u/1 -> Integer Delay/1, Integer Delay/2, Add/2
  Integer Delay/1 -> Add/1
  Gain6/1 -> du/dt/1

== system SimForces2020a/sbVDCController/sbFormTotalRequiredForces/sbTotalRequiredForcesPS2/sbFilteredVelocityDerivativeP22/sbDiscreteDerivative2 ==
  u : Inport
  Add : Sum  Inputs=-+
  Gain6 : Gain  Gain=1/(2*controller.dT)
  Integer Delay : Delay  InitialConditionSource=Input port  InitialCondition=0  SampleTime=controller.dT
      settings: InputPortMap=u0,p4
  du/dt : Outport  PortDimensions=1
  wires:
  u/1 -> Integer Delay/1, Integer Delay/2, Add/2
  Integer Delay/1 -> Add/1
  Add/1 -> Gain6/1
  Gain6/1 -> du/dt/1

== system SimForces2020a/sbVDCController/sbFormTotalRequiredForces/sbTotalRequiredForcesPS2/sbFilteredVelocityDerivativeP22/sbDiscreteDerivative3 ==
  u : Inport
  Add : Sum  Inputs=-+
  Gain6 : Gain  Gain=1/(2*controller.dT)
  Integer Delay : Delay  InitialConditionSource=Input port  InitialCondition=0  SampleTime=controller.dT
      settings: InputPortMap=u0,p4
  du/dt : Outport  PortDimensions=1
  wires:
  Add/1 -> Gain6/1
  Integer Delay/1 -> Add/1
  u/1 -> Integer Delay/1, Integer Delay/2, Add/2
  Gain6/1 -> du/dt/1

== system SimForces2020a/sbVDCController/sbFormTotalRequiredForces/sbTotalRequiredForcesPS2/sbFilteredVelocityDerivativeP22/sbDiscreteDerivative4 ==
  u : Inport
  Add : Sum  Inputs=-+
  Gain6 : Gain  Gain=1/(2*controller.dT)
  Integer Delay : Delay  InitialConditionSource=Input port  InitialCondition=0  SampleTime=controller.dT
      settings: InputPortMap=u0,p4
  du/dt : Outport  PortDimensions=1
  wires:
  Add/1 -> Gain6/1
  Integer Delay/1 -> Add/1
  u/1 -> Integer Delay/1, Integer Delay/2, Add/2
  Gain6/1 -> du/dt/1

== system SimForces2020a/sbVDCController/sbFormTotalRequiredForces/sbTotalRequiredForcesPS2/sbFilteredVelocityDerivativeP22/sbDiscreteDerivative5 ==
  u : Inport
  Add : Sum  Inputs=-+
  Gain6 : Gain  Gain=1/(2*controller.dT)
  Integer Delay : Delay  InitialConditionSource=Input port  InitialCondition=0  SampleTime=controller.dT
      settings: InputPortMap=u0,p4
  du/dt : Outport  PortDimensions=1
  wires:
  Add/1 -> Gain6/1
  Integer Delay/1 -> Add/1
  u/1 -> Integer Delay/1, Integer Delay/2, Add/2
  Gain6/1 -> du/dt/1

== system SimForces2020a/sbVDCController/sbFormTotalRequiredForces/sbTotalRequiredForcesPS2/sbFilteredVelocityDerivativeP22/sbDiscreteDerivative6 ==
  u : Inport
  Add : Sum  Inputs=-+
  Gain6 : Gain  Gain=1/(2*controller.dT)
  Integer Delay : Delay  InitialConditionSource=Input port  InitialCondition=0  SampleTime=controller.dT
      settings: InputPortMap=u0,p4
  du/dt : Outport  PortDimensions=1
  wires:
  Add/1 -> Gain6/1
  Integer Delay/1 -> Add/1
  u/1 -> Integer Delay/1, Integer Delay/2, Add/2
  Gain6/1 -> du/dt/1

== system SimForces2020a/sbVDCController/sbFormTotalRequiredForces/sbTotalRequiredForcesPS2/sbFilteredVelocityDerivativeP22/sbLowPassFilter1 ==
  dV : Inport
  Delay : Delay  InitialConditionSource=Input port  SampleTime=filtDV.dT
      settings: InputPortMap=u0,p4
  Delay1 : Delay  DelayLength=1  InitialConditionSource=Input port  SampleTime=filtDV.dT
      settings: InputPortMap=u0,p4
  Delay2 : Delay  DelayLength=0  InitialConditionSource=Input port  SampleTime=filtDV.dT
      settings: InputPortMap=u0,p4
  Delay3 : Delay  InitialConditionSource=Input port  SampleTime=filtDV.dT
      settings: InputPortMap=u0,p4
  Delay4 : Delay  DelayLength=1  InitialConditionSource=Input port  SampleTime=filtDV.dT
      settings: InputPortMap=u0,p4
  Gain : Gain  Gain=filtDV.a0
  Gain1 : Gain  Gain=filtDV.b1
  Gain2 : Gain  Gain=filtDV.b2
  Gain3 : Gain  Gain=filtDV.b0
  Gain4 : Gain  Gain=filtDV.a1
  Sum : Sum  Inputs=|--+++
  dVFilt : Outport
  wires:
  Gain3/1 -> Sum/5
  Gain2/1 -> Sum/3
  Delay4/1 -> Gain4/1
  Delay/1 -> Gain/1
  Delay1/1 -> Gain1/1
  Delay2/1 -> Gain2/1
  Gain4/1 -> Sum/1
  Sum/1 -> dVFilt/1, Delay4/1, Delay/1  "dVFilt"
  dV/1 -> Delay2/1, Delay2/2, Delay1/1, Delay3/2, Delay3/1, Delay1/2, Delay4/2, Delay/2  "dV"
  Gain1/1 -> Sum/4
  Gain/1 -> Sum/2
  Delay3/1 -> Gain3/1

== system SimForces2020a/sbVDCController/sbFormTotalRequiredForces/sbTotalRequiredForcesPS2/sbFilteredVelocityDerivativeP22/sbLowPassFilter2 ==
  dV : Inport
  Delay : Delay  InitialConditionSource=Input port  SampleTime=filtDV.dT
      settings: InputPortMap=u0,p4
  Delay1 : Delay  DelayLength=1  InitialConditionSource=Input port  SampleTime=filtDV.dT
      settings: InputPortMap=u0,p4
  Delay2 : Delay  DelayLength=0  InitialConditionSource=Input port  SampleTime=filtDV.dT
      settings: InputPortMap=u0,p4
  Delay3 : Delay  InitialConditionSource=Input port  SampleTime=filtDV.dT
      settings: InputPortMap=u0,p4
  Delay4 : Delay  DelayLength=1  InitialConditionSource=Input port  SampleTime=filtDV.dT
      settings: InputPortMap=u0,p4
  Gain : Gain  Gain=filtDV.a0
  Gain1 : Gain  Gain=filtDV.b1
  Gain2 : Gain  Gain=filtDV.b2
  Gain3 : Gain  Gain=filtDV.b0
  Gain4 : Gain  Gain=filtDV.a1
  Sum : Sum  Inputs=|--+++
  dVFilt : Outport
  wires:
  Delay3/1 -> Gain3/1
  Gain/1 -> Sum/2
  Gain1/1 -> Sum/4
  dV/1 -> Delay/2, Delay4/2, Delay1/2, Delay3/1, Delay3/2, Delay1/1, Delay2/2, Delay2/1  "dV"
  Sum/1 -> Delay/1, Delay4/1, dVFilt/1  "dVFilt"
  Gain4/1 -> Sum/1
  Delay2/1 -> Gain2/1
  Delay1/1 -> Gain1/1
  Delay/1 -> Gain/1
  Delay4/1 -> Gain4/1
  Gain2/1 -> Sum/3
  Gain3/1 -> Sum/5

== system SimForces2020a/sbVDCController/sbFormTotalRequiredForces/sbTotalRequiredForcesPS2/sbFilteredVelocityDerivativeP22/sbLowPassFilter3 ==
  dV : Inport
  Delay : Delay  InitialConditionSource=Input port  SampleTime=filtDV.dT
      settings: InputPortMap=u0,p4
  Delay1 : Delay  DelayLength=1  InitialConditionSource=Input port  SampleTime=filtDV.dT
      settings: InputPortMap=u0,p4
  Delay2 : Delay  DelayLength=0  InitialConditionSource=Input port  SampleTime=filtDV.dT
      settings: InputPortMap=u0,p4
  Delay3 : Delay  InitialConditionSource=Input port  SampleTime=filtDV.dT
      settings: InputPortMap=u0,p4
  Delay4 : Delay  DelayLength=1  InitialConditionSource=Input port  SampleTime=filtDV.dT
      settings: InputPortMap=u0,p4
  Gain : Gain  Gain=filtDV.a0
  Gain1 : Gain  Gain=filtDV.b1
  Gain2 : Gain  Gain=filtDV.b2
  Gain3 : Gain  Gain=filtDV.b0
  Gain4 : Gain  Gain=filtDV.a1
  Sum : Sum  Inputs=|--+++
  dVFilt : Outport
  wires:
  Gain3/1 -> Sum/5
  Gain2/1 -> Sum/3
  Delay4/1 -> Gain4/1
  Delay/1 -> Gain/1
  Delay1/1 -> Gain1/1
  Delay2/1 -> Gain2/1
  Gain4/1 -> Sum/1
  Sum/1 -> dVFilt/1, Delay4/1, Delay/1  "dVFilt"
  dV/1 -> Delay2/1, Delay2/2, Delay1/1, Delay3/2, Delay3/1, Delay1/2, Delay4/2, Delay/2  "dV"
  Gain1/1 -> Sum/4
  Gain/1 -> Sum/2
  Delay3/1 -> Gain3/1

== system SimForces2020a/sbVDCController/sbFormTotalRequiredForces/sbTotalRequiredForcesPS2/sbFilteredVelocityDerivativeP22/sbLowPassFilter4 ==
  dV : Inport
  Delay : Delay  InitialConditionSource=Input port  SampleTime=filtDV.dT
      settings: InputPortMap=u0,p4
  Delay1 : Delay  DelayLength=1  InitialConditionSource=Input port  SampleTime=filtDV.dT
      settings: InputPortMap=u0,p4
  Delay2 : Delay  DelayLength=0  InitialConditionSource=Input port  SampleTime=filtDV.dT
      settings: InputPortMap=u0,p4
  Delay3 : Delay  InitialConditionSource=Input port  SampleTime=filtDV.dT
      settings: InputPortMap=u0,p4
  Delay4 : Delay  DelayLength=1  InitialConditionSource=Input port  SampleTime=filtDV.dT
      settings: InputPortMap=u0,p4
  Gain : Gain  Gain=filtDV.a0
  Gain1 : Gain  Gain=filtDV.b1
  Gain2 : Gain  Gain=filtDV.b2
  Gain3 : Gain  Gain=filtDV.b0
  Gain4 : Gain  Gain=filtDV.a1
  Sum : Sum  Inputs=|--+++
  dVFilt : Outport
  wires:
  Delay3/1 -> Gain3/1
  Gain/1 -> Sum/2
  Gain1/1 -> Sum/4
  dV/1 -> Delay/2, Delay4/2, Delay1/2, Delay3/1, Delay3/2, Delay1/1, Delay2/2, Delay2/1  "dV"
  Sum/1 -> Delay/1, Delay4/1, dVFilt/1  "dVFilt"
  Gain4/1 -> Sum/1
  Delay2/1 -> Gain2/1
  Delay1/1 -> Gain1/1
  Delay/1 -> Gain/1
  Delay4/1 -> Gain4/1
  Gain2/1 -> Sum/3
  Gain3/1 -> Sum/5

== system SimForces2020a/sbVDCController/sbFormTotalRequiredForces/sbTotalRequiredForcesPS2/sbFilteredVelocityDerivativeP22/sbLowPassFilter5 ==
  dV : Inport
  Delay : Delay  InitialConditionSource=Input port  SampleTime=filtDV.dT
      settings: InputPortMap=u0,p4
  Delay1 : Delay  DelayLength=1  InitialConditionSource=Input port  SampleTime=filtDV.dT
      settings: InputPortMap=u0,p4
  Delay2 : Delay  DelayLength=0  InitialConditionSource=Input port  SampleTime=filtDV.dT
      settings: InputPortMap=u0,p4
  Delay3 : Delay  InitialConditionSource=Input port  SampleTime=filtDV.dT
      settings: InputPortMap=u0,p4
  Delay4 : Delay  DelayLength=1  InitialConditionSource=Input port  SampleTime=filtDV.dT
      settings: InputPortMap=u0,p4
  Gain : Gain  Gain=filtDV.a0
  Gain1 : Gain  Gain=filtDV.b1
  Gain2 : Gain  Gain=filtDV.b2
  Gain3 : Gain  Gain=filtDV.b0
  Gain4 : Gain  Gain=filtDV.a1
  Sum : Sum  Inputs=|--+++
  dVFilt : Outport
  wires:
  Gain3/1 -> Sum/5
  Gain2/1 -> Sum/3
  Delay4/1 -> Gain4/1
  Delay/1 -> Gain/1
  Delay1/1 -> Gain1/1
  Delay2/1 -> Gain2/1
  Gain4/1 -> Sum/1
  Sum/1 -> dVFilt/1, Delay4/1, Delay/1  "dVFilt"
  dV/1 -> Delay2/1, Delay2/2, Delay1/1, Delay3/2, Delay3/1, Delay1/2, Delay4/2, Delay/2  "dV"
  Gain1/1 -> Sum/4
  Gain/1 -> Sum/2
  Delay3/1 -> Gain3/1

== system SimForces2020a/sbVDCController/sbFormTotalRequiredForces/sbTotalRequiredForcesPS2/sbFilteredVelocityDerivativeP22/sbLowPassFilter6 ==
  dV : Inport
  Delay : Delay  InitialConditionSource=Input port  SampleTime=filtDV.dT
      settings: InputPortMap=u0,p4
  Delay1 : Delay  DelayLength=1  InitialConditionSource=Input port  SampleTime=filtDV.dT
      settings: InputPortMap=u0,p4
  Delay2 : Delay  DelayLength=0  InitialConditionSource=Input port  SampleTime=filtDV.dT
      settings: InputPortMap=u0,p4
  Delay3 : Delay  InitialConditionSource=Input port  SampleTime=filtDV.dT
      settings: InputPortMap=u0,p4
  Delay4 : Delay  DelayLength=1  InitialConditionSource=Input port  SampleTime=filtDV.dT
      settings: InputPortMap=u0,p4
  Gain : Gain  Gain=filtDV.a0
  Gain1 : Gain  Gain=filtDV.b1
  Gain2 : Gain  Gain=filtDV.b2
  Gain3 : Gain  Gain=filtDV.b0
  Gain4 : Gain  Gain=filtDV.a1
  Sum : Sum  Inputs=|--+++
  dVFilt : Outport
  wires:
  Delay3/1 -> Gain3/1
  Gain/1 -> Sum/2
  Gain1/1 -> Sum/4
  dV/1 -> Delay/2, Delay4/2, Delay1/2, Delay3/1, Delay3/2, Delay1/1, Delay2/2, Delay2/1  "dV"
  Sum/1 -> Delay/1, Delay4/1, dVFilt/1  "dVFilt"
  Gain4/1 -> Sum/1
  Delay2/1 -> Gain2/1
  Delay1/1 -> Gain1/1
  Delay/1 -> Gain/1
  Delay4/1 -> Gain4/1
  Gain2/1 -> Sum/3
  Gain3/1 -> Sum/5

== system SimForces2020a/sbVDCController/sbFormTotalRequiredForces/sbTotalRequiredForcesPS2/sbFilteredVelocityDerivativeP32/sbDiscreteDerivative1 ==
  u : Inport
  Add : Sum  Inputs=-+
  Gain6 : Gain  Gain=1/(2*controller.dT)
  Integer Delay : Delay  InitialConditionSource=Input port  InitialCondition=0  SampleTime=controller.dT
      settings: InputPortMap=u0,p4
  du/dt : Outport  PortDimensions=1
  wires:
  Add/1 -> Gain6/1
  u/1 -> Integer Delay/1, Integer Delay/2, Add/2
  Integer Delay/1 -> Add/1
  Gain6/1 -> du/dt/1

== system SimForces2020a/sbVDCController/sbFormTotalRequiredForces/sbTotalRequiredForcesPS2/sbFilteredVelocityDerivativeP32/sbDiscreteDerivative2 ==
  u : Inport
  Add : Sum  Inputs=-+
  Gain6 : Gain  Gain=1/(2*controller.dT)
  Integer Delay : Delay  InitialConditionSource=Input port  InitialCondition=0  SampleTime=controller.dT
      settings: InputPortMap=u0,p4
  du/dt : Outport  PortDimensions=1
  wires:
  u/1 -> Integer Delay/1, Integer Delay/2, Add/2
  Integer Delay/1 -> Add/1
  Add/1 -> Gain6/1
  Gain6/1 -> du/dt/1

== system SimForces2020a/sbVDCController/sbFormTotalRequiredForces/sbTotalRequiredForcesPS2/sbFilteredVelocityDerivativeP32/sbDiscreteDerivative3 ==
  u : Inport
  Add : Sum  Inputs=-+
  Gain6 : Gain  Gain=1/(2*controller.dT)
  Integer Delay : Delay  InitialConditionSource=Input port  InitialCondition=0  SampleTime=controller.dT
      settings: InputPortMap=u0,p4
  du/dt : Outport  PortDimensions=1
  wires:
  Add/1 -> Gain6/1
  Integer Delay/1 -> Add/1
  u/1 -> Integer Delay/1, Integer Delay/2, Add/2
  Gain6/1 -> du/dt/1

== system SimForces2020a/sbVDCController/sbFormTotalRequiredForces/sbTotalRequiredForcesPS2/sbFilteredVelocityDerivativeP32/sbDiscreteDerivative4 ==
  u : Inport
  Add : Sum  Inputs=-+
  Gain6 : Gain  Gain=1/(2*controller.dT)
  Integer Delay : Delay  InitialConditionSource=Input port  InitialCondition=0  SampleTime=controller.dT
      settings: InputPortMap=u0,p4
  du/dt : Outport  PortDimensions=1
  wires:
  Add/1 -> Gain6/1
  Integer Delay/1 -> Add/1
  u/1 -> Integer Delay/1, Integer Delay/2, Add/2
  Gain6/1 -> du/dt/1

== system SimForces2020a/sbVDCController/sbFormTotalRequiredForces/sbTotalRequiredForcesPS2/sbFilteredVelocityDerivativeP32/sbDiscreteDerivative5 ==
  u : Inport
  Add : Sum  Inputs=-+
  Gain6 : Gain  Gain=1/(2*controller.dT)
  Integer Delay : Delay  InitialConditionSource=Input port  InitialCondition=0  SampleTime=controller.dT
      settings: InputPortMap=u0,p4
  du/dt : Outport  PortDimensions=1
  wires:
  Add/1 -> Gain6/1
  Integer Delay/1 -> Add/1
  u/1 -> Integer Delay/1, Integer Delay/2, Add/2
  Gain6/1 -> du/dt/1

== system SimForces2020a/sbVDCController/sbFormTotalRequiredForces/sbTotalRequiredForcesPS2/sbFilteredVelocityDerivativeP32/sbDiscreteDerivative6 ==
  u : Inport
  Add : Sum  Inputs=-+
  Gain6 : Gain  Gain=1/(2*controller.dT)
  Integer Delay : Delay  InitialConditionSource=Input port  InitialCondition=0  SampleTime=controller.dT
      settings: InputPortMap=u0,p4
  du/dt : Outport  PortDimensions=1
  wires:
  Add/1 -> Gain6/1
  Integer Delay/1 -> Add/1
  u/1 -> Integer Delay/1, Integer Delay/2, Add/2
  Gain6/1 -> du/dt/1

== system SimForces2020a/sbVDCController/sbFormTotalRequiredForces/sbTotalRequiredForcesPS2/sbFilteredVelocityDerivativeP32/sbLowPassFilter1 ==
  dV : Inport
  Delay : Delay  InitialConditionSource=Input port  SampleTime=filtDV.dT
      settings: InputPortMap=u0,p4
  Delay1 : Delay  DelayLength=1  InitialConditionSource=Input port  SampleTime=filtDV.dT
      settings: InputPortMap=u0,p4
  Delay2 : Delay  DelayLength=0  InitialConditionSource=Input port  SampleTime=filtDV.dT
      settings: InputPortMap=u0,p4
  Delay3 : Delay  InitialConditionSource=Input port  SampleTime=filtDV.dT
      settings: InputPortMap=u0,p4
  Delay4 : Delay  DelayLength=1  InitialConditionSource=Input port  SampleTime=filtDV.dT
      settings: InputPortMap=u0,p4
  Gain : Gain  Gain=filtDV.a0
  Gain1 : Gain  Gain=filtDV.b1
  Gain2 : Gain  Gain=filtDV.b2
  Gain3 : Gain  Gain=filtDV.b0
  Gain4 : Gain  Gain=filtDV.a1
  Sum : Sum  Inputs=|--+++
  dVFilt : Outport
  wires:
  Gain3/1 -> Sum/5
  Gain2/1 -> Sum/3
  Delay4/1 -> Gain4/1
  Delay/1 -> Gain/1
  Delay1/1 -> Gain1/1
  Delay2/1 -> Gain2/1
  Gain4/1 -> Sum/1
  Sum/1 -> dVFilt/1, Delay4/1, Delay/1  "dVFilt"
  dV/1 -> Delay2/1, Delay2/2, Delay1/1, Delay3/2, Delay3/1, Delay1/2, Delay4/2, Delay/2  "dV"
  Gain1/1 -> Sum/4
  Gain/1 -> Sum/2
  Delay3/1 -> Gain3/1

== system SimForces2020a/sbVDCController/sbFormTotalRequiredForces/sbTotalRequiredForcesPS2/sbFilteredVelocityDerivativeP32/sbLowPassFilter2 ==
  dV : Inport
  Delay : Delay  InitialConditionSource=Input port  SampleTime=filtDV.dT
      settings: InputPortMap=u0,p4
  Delay1 : Delay  DelayLength=1  InitialConditionSource=Input port  SampleTime=filtDV.dT
      settings: InputPortMap=u0,p4
  Delay2 : Delay  DelayLength=0  InitialConditionSource=Input port  SampleTime=filtDV.dT
      settings: InputPortMap=u0,p4
  Delay3 : Delay  InitialConditionSource=Input port  SampleTime=filtDV.dT
      settings: InputPortMap=u0,p4
  Delay4 : Delay  DelayLength=1  InitialConditionSource=Input port  SampleTime=filtDV.dT
      settings: InputPortMap=u0,p4
  Gain : Gain  Gain=filtDV.a0
  Gain1 : Gain  Gain=filtDV.b1
  Gain2 : Gain  Gain=filtDV.b2
  Gain3 : Gain  Gain=filtDV.b0
  Gain4 : Gain  Gain=filtDV.a1
  Sum : Sum  Inputs=|--+++
  dVFilt : Outport
  wires:
  Delay3/1 -> Gain3/1
  Gain/1 -> Sum/2
  Gain1/1 -> Sum/4
  dV/1 -> Delay/2, Delay4/2, Delay1/2, Delay3/1, Delay3/2, Delay1/1, Delay2/2, Delay2/1  "dV"
  Sum/1 -> Delay/1, Delay4/1, dVFilt/1  "dVFilt"
  Gain4/1 -> Sum/1
  Delay2/1 -> Gain2/1
  Delay1/1 -> Gain1/1
  Delay/1 -> Gain/1
  Delay4/1 -> Gain4/1
  Gain2/1 -> Sum/3
  Gain3/1 -> Sum/5

== system SimForces2020a/sbVDCController/sbFormTotalRequiredForces/sbTotalRequiredForcesPS2/sbFilteredVelocityDerivativeP32/sbLowPassFilter3 ==
  dV : Inport
  Delay : Delay  InitialConditionSource=Input port  SampleTime=filtDV.dT
      settings: InputPortMap=u0,p4
  Delay1 : Delay  DelayLength=1  InitialConditionSource=Input port  SampleTime=filtDV.dT
      settings: InputPortMap=u0,p4
  Delay2 : Delay  DelayLength=0  InitialConditionSource=Input port  SampleTime=filtDV.dT
      settings: InputPortMap=u0,p4
  Delay3 : Delay  InitialConditionSource=Input port  SampleTime=filtDV.dT
      settings: InputPortMap=u0,p4
  Delay4 : Delay  DelayLength=1  InitialConditionSource=Input port  SampleTime=filtDV.dT
      settings: InputPortMap=u0,p4
  Gain : Gain  Gain=filtDV.a0
  Gain1 : Gain  Gain=filtDV.b1
  Gain2 : Gain  Gain=filtDV.b2
  Gain3 : Gain  Gain=filtDV.b0
  Gain4 : Gain  Gain=filtDV.a1
  Sum : Sum  Inputs=|--+++
  dVFilt : Outport
  wires:
  Gain3/1 -> Sum/5
  Gain2/1 -> Sum/3
  Delay4/1 -> Gain4/1
  Delay/1 -> Gain/1
  Delay1/1 -> Gain1/1
  Delay2/1 -> Gain2/1
  Gain4/1 -> Sum/1
  Sum/1 -> dVFilt/1, Delay4/1, Delay/1  "dVFilt"
  dV/1 -> Delay2/1, Delay2/2, Delay1/1, Delay3/2, Delay3/1, Delay1/2, Delay4/2, Delay/2  "dV"
  Gain1/1 -> Sum/4
  Gain/1 -> Sum/2
  Delay3/1 -> Gain3/1
